simulink model "uniciclo_FL2"  (R2020a)
settings: Solver=VariableStepAuto  StartTime=0.0  StopTime=Inf  MaxStep=0.01  RelTol=1e-3
InitFcn:
  | init_biciclo
StopFcn:
  | stop_uniciclo
values from neighbouring files (symbols this model uses):
  L = 1    [init_biciclo.m]
  phi_iniziale = 0    [init_biciclo.m]
  theta_P_iniziale = pi/3    (= 1.0471975512)    [init_biciclo.m]
  v_P_dot_iniziale = 0    [init_biciclo.m]
  v_P_iniziale = 1    [init_biciclo.m]
  x_M_iniziale = 10    [init_biciclo.m]
  y_M_iniziale = -20    [init_biciclo.m]
undefined symbols (not defined in the file or in its folder): a, indexclot, Lsofar, Lsofarclot, n_p, s_f, t_f, theta_rette, v, v_raggiunta, xp, yp
libraries: simulink x1
settings Model: Creator=Andrea_Ferroni  LastModifiedBy=Andrea_Ferroni

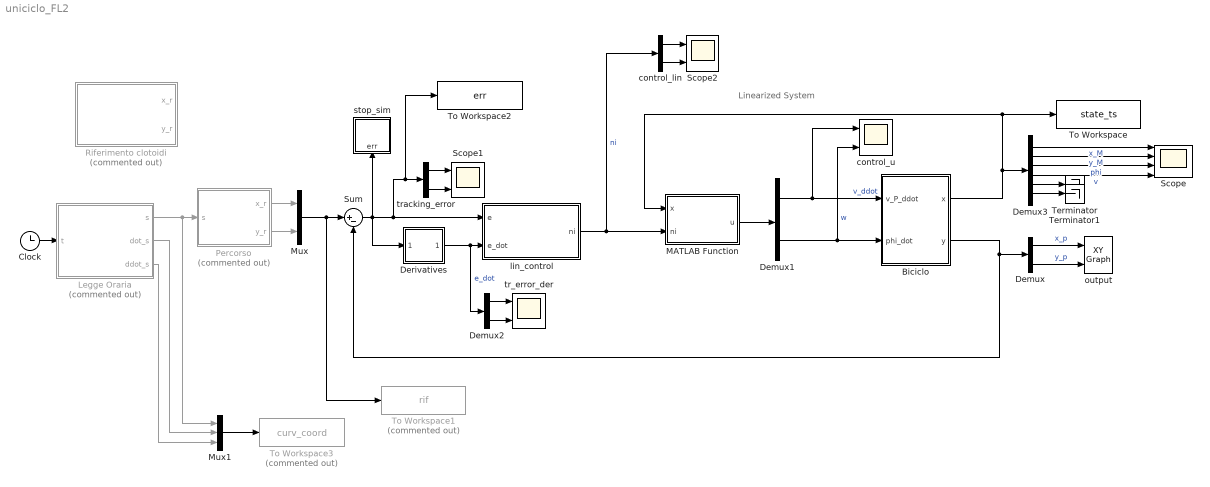
== system uniciclo_FL2 ==
  note: Linearized System
  Biciclo : Subsystem
  Clock : Clock
  Demux : Demux  Outputs=2
  Demux1 : Demux  Outputs=2
  Demux2 : Demux  Outputs=2
  Demux3 : Demux  Outputs=6
  Derivatives : Subsystem
  Legge Oraria : MATLAB Function  Commented=on  TreatAsAtomicUnit=on
  MATLAB Function : MATLAB Function  TreatAsAtomicUnit=on
  Mux : Mux  Inputs=2
  Mux1 : Mux  Inputs=3
  Percorso : MATLAB Function  Commented=on  TreatAsAtomicUnit=on
  Riferimento clotoidi : Subsystem  Commented=on
  Scope : Scope  NumInputPorts=4
  Scope1 : Scope  NumInputPorts=2
  Scope2 : Scope  NumInputPorts=2
  Sum : Sum  Inputs=|+-
  Terminator : Terminator
  Terminator1 : Terminator
  To Workspace : ToWorkspace  VariableName=state_ts  SaveFormat=Timeseries  SampleTime=-1
  To Workspace1 : ToWorkspace  Commented=on  VariableName=rif  SaveFormat=Timeseries  SampleTime=-1
  To Workspace2 : ToWorkspace  VariableName=err  SaveFormat=Timeseries  SampleTime=-1
  To Workspace3 : ToWorkspace  Commented=on  VariableName=curv_coord  SaveFormat=Timeseries  SampleTime=-1
  control_lin : Demux  Outputs=2
  control_u : Scope  NumInputPorts=2
  lin_control : MATLAB Function  TreatAsAtomicUnit=on
  output : simulink/Sinks/XY Graph  xmin=-50  xmax=50  ymin=-50  ymax=50  st=-1
  stop_sim : Subsystem
  tr_error_der : Scope  NumInputPorts=2
  tracking_error : Demux  Outputs=2
  wires:
  Biciclo/1(x) -> To Workspace/1, MATLAB Function/1(x), Demux3/1
  Mux/1 -> Sum/1, To Workspace1/1
  Biciclo/2(y) -> Demux/1, Sum/2
  lin_control/1(ni) -> control_lin/1, MATLAB Function/2(ni)  "ni"
  Sum/1 -> Derivatives/1(In1), lin_control/1(e), To Workspace2/1, tracking_error/1, stop_sim/1(err)
  Derivatives/1(Out1) -> Demux2/1, lin_control/2(e_dot)  "e_dot"
  Demux/1 -> output/1  "x_p"
  Demux/2 -> output/2  "y_p"
  Demux2/1 -> tr_error_der/1
  Demux2/2 -> tr_error_der/2
  tracking_error/1 -> Scope1/1
  tracking_error/2 -> Scope1/2
  MATLAB Function/1(u) -> Demux1/1
  Demux1/1 -> control_u/1, Biciclo/1(v_P_ddot)  "v_ddot"
  Demux1/2 -> control_u/2, Biciclo/2(phi_dot)  "w"
  control_lin/2 -> Scope2/2
  control_lin/1 -> Scope2/1
  Demux3/1 -> Scope/1  "x_M"
  Demux3/2 -> Scope/2  "y_M"
  Demux3/3 -> Scope/3  "phi"
  Demux3/4 -> Scope/4  "v"
  Clock/1 -> Legge Oraria/1(t)
  Legge Oraria/1(s) -> Mux1/1, Percorso/1(s)
  Percorso/1(x_r) -> Mux/1
  Percorso/2(y_r) -> Mux/2
  Mux1/1 -> To Workspace3/1
  Legge Oraria/3(ddot_s) -> Mux1/3
  Legge Oraria/2(dot_s) -> Mux1/2
  Demux3/6 -> Terminator1/1
  Demux3/5 -> Terminator/1

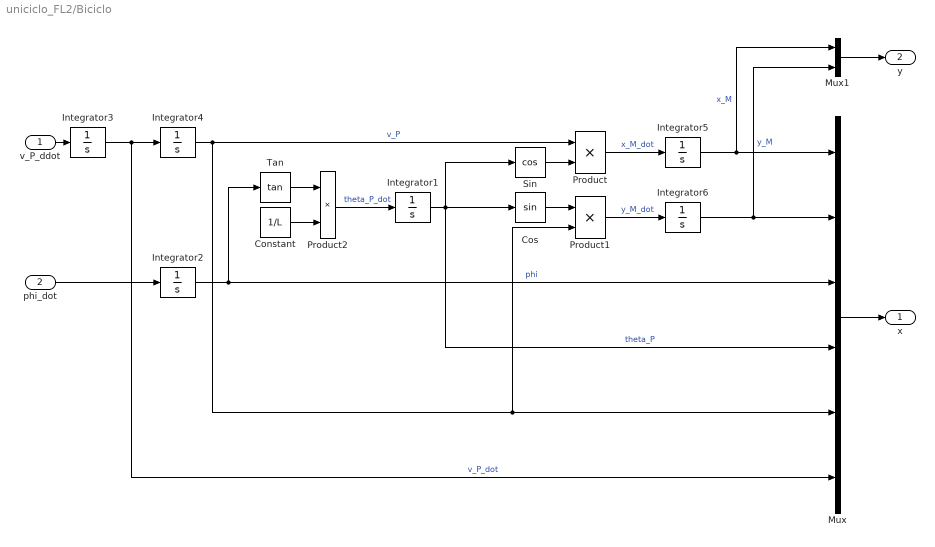
== system uniciclo_FL2/Biciclo ==
  v_P_ddot : Inport
  phi_dot : Inport  Port=2
  Constant : Constant  Value=1/L
  Cos : Trigonometry
  Integrator1 : Integrator  InitialCondition=theta_P_iniziale
  Integrator2 : Integrator  InitialCondition=phi_iniziale
  Integrator3 : Integrator  InitialCondition=v_P_dot_iniziale
  Integrator4 : Integrator  InitialCondition=v_P_iniziale
  Integrator5 : Integrator  InitialCondition=x_M_iniziale
  Integrator6 : Integrator  InitialCondition=y_M_iniziale
  Mux : Mux  Inputs=6
  Mux1 : Mux  Inputs=2
  Product : Product
  Product1 : Product
  Product2 : Product
  Sin : Trigonometry  Operator=cos
  Tan : Trigonometry  Operator=tan
  x : Outport
  y : Outport  Port=2
  wires:
  v_P_ddot/1 -> Integrator3/1
  phi_dot/1 -> Integrator2/1
  Mux/1 -> x/1
  Integrator3/1 -> Integrator4/1, Mux/6  "v_P_dot"
  Integrator1/1 -> Sin/1, Mux/4, Cos/1  "theta_P"
  Integrator4/1 -> Product1/2, Mux/5, Product/1  "v_P"
  Integrator2/1 -> Tan/1, Mux/3  "phi"
  Sin/1 -> Product/2
  Cos/1 -> Product1/1
  Product/1 -> Integrator5/1  "x_M_dot"
  Product1/1 -> Integrator6/1  "y_M_dot"
  Tan/1 -> Product2/1
  Constant/1 -> Product2/2
  Product2/1 -> Integrator1/1  "theta_P_dot"
  Mux1/1 -> y/1
  Integrator5/1 -> Mux1/1, Mux/1  "x_M"
  Integrator6/1 -> Mux1/2, Mux/2  "y_M"

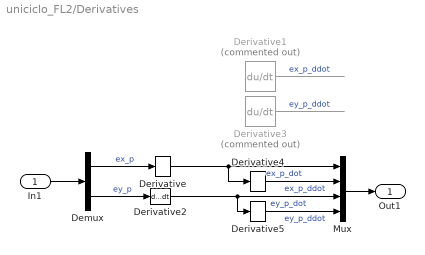
== system uniciclo_FL2/Derivatives ==
  In1 : Inport
  Demux : Demux  Outputs=2
  Derivative{,2,4..5} (4 alike) : Derivative  CoefficientInTFapproximation=1e10
  Derivative1 : Derivative  Commented=on  CoefficientInTFapproximation=1e10
  Derivative3 : Derivative  Commented=on  CoefficientInTFapproximation=1e10
  Mux : Mux
  Out1 : Outport
  wires:
  In1/1 -> Demux/1
  Demux/1 -> Derivative/1  "ex_p"
  Derivative/1 -> Derivative4/1, Mux/1  "ex_p_dot"
  Demux/2 -> Derivative2/1  "ey_p"
  Derivative1/1 -> ?  "ex_p_ddot"
  Derivative3/1 -> ?  "ey_p_ddot"
  Mux/1 -> Out1/1
  Derivative4/1 -> Mux/2  "ex_p_ddot"
  Derivative2/1 -> Derivative5/1, Mux/3  "ey_p_dot"
  Derivative5/1 -> Mux/4  "ey_p_ddot"

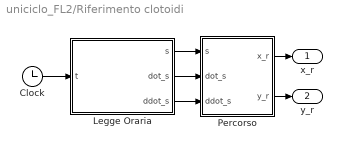
== system uniciclo_FL2/Riferimento clotoidi ==
  Clock : Clock
  Legge Oraria : MATLAB Function  TreatAsAtomicUnit=on
  Percorso : MATLAB Function  TreatAsAtomicUnit=on
  x_r : Outport
  y_r : Outport  Port=2
  wires:
  Clock/1 -> Legge Oraria/1(t)
  Legge Oraria/2(dot_s) -> Percorso/2(dot_s)
  Legge Oraria/1(s) -> Percorso/1(s)
  Legge Oraria/3(ddot_s) -> Percorso/3(ddot_s)
  Percorso/1(x_r) -> x_r/1
  Percorso/2(y_r) -> y_r/1

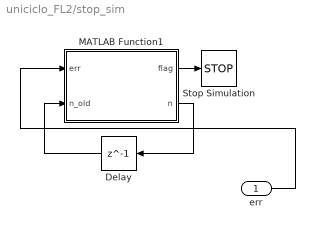
== system uniciclo_FL2/stop_sim ==
  err : Inport
  Delay : Delay  DelayLength=1
  MATLAB Function1 : MATLAB Function  TreatAsAtomicUnit=on
  Stop Simulation : Stop
  wires:
  MATLAB Function1/2(n) -> Delay/1
  MATLAB Function1/1(flag) -> Stop Simulation/1
  err/1 -> MATLAB Function1/1(err)
  Delay/1 -> MATLAB Function1/2(n_old)

== matlab function uniciclo_FL2/lin_control ==
  data: e input; ni output; e_dot input
function ni = lin_control(e, e_dot)%, K1, K2

% ni = K1.*e + K2.*e_dot;

ni = [0;0];
end

== matlab function uniciclo_FL2/MATLAB Function ==
  data: x input; ni input; u output; L parameter
function u = Linearized(x,ni,L)
E_inv = inv_E(x,L);
G = Gamma(x,L);
u =  -E_inv*G + E_inv*ni;
end

% gamma
function Gm = Gamma(x,L)
phi = x(3);
theta_P = x(4);
v_P = x(5);
v_dot = x(6);
Gm = [- (v_P*tan(phi)*((cos(theta_P)*tan(phi)*v_P^2)/L + v_dot*sin(theta_P)))/L - (2*v_P*v_dot*tan(phi)*sin(theta_P))/L;...
		(v_P*tan(phi)*(v_dot*cos(theta_P) - (v_P^2*tan(phi)*sin(theta_P))/L))/L + (2*v_P*v_dot*cos(theta_P)*tan(phi))/L];
end
% 
function E_in = inv_E(x,L)
phi = x(3);
theta_P = x(4);
v_P = x(5);
E =[ cos(theta_P), -(v_P^2*sin(theta_P)*(tan(phi)^2 + 1))/L;...
    sin(theta_P),  (v_P^2*cos(theta_P)*(tan(phi)^2 + 1))/L];
E_in = inv(E);
end

== matlab function uniciclo_FL2/Riferimento clotoidi/Legge Oraria ==
  data: t input; s output; dot_s output; ddot_s output; v_iniziale parameter
function [s, dot_s, ddot_s] = legge_oraria(t,v_iniziale)
%#codegen PEPO

s = v_iniziale*t;
dot_s = v_iniziale;
ddot_s = 0.0;

%     if v_raggiunta==0
%         
%         if t<=(s_f/a)^0.5               %acce
%             s= 0.5*a*t^2;
%             dot_s=a*t;
%             ddot_s=a;
%             
%         elseif t>(s_f/a)^0.5 & t<=t_f   %decel
%             s=s_f-0.5*a*(t_f-t)^2;
%             dot_s=-a*t;
%             ddot_s=-a;
%             
%         end
%     
%     else    
%         
%         if t<=v/a                       %acc
%             s=0.5*a*t^2;
%             dot_s=a*t;
%             ddot_s=a;
%             
%         elseif t>v/a & t<=t_f-v/a       %v=cost
%             s=0.5*a*(v/a)^2 + v *(t-v/a);
%             dot_s=v;
%             ddot_s=0;
%             
%         elseif t>t_f-v/a & t<=t_f       %decel
%             s=s_f-0.5*a*(t_f-t)^2;
%             dot_s=v-a*(t - (t_f-v/a));
%             ddot_s=-a;
%             
%             
%         end
%             
%     end

end

== matlab function uniciclo_FL2/stop_sim/MATLAB Function1 ==
  data: flag output; err input; n output; n_old input; threshold parameter
function [flag, n] = stop_function(err, n_old, threshold)
	flag = 0;
	n = n_old;
	if norm(err, 2) < threshold
		n=n+1;
	else
		n=0;
	end
	
	if n > 10
		flag = 1;
		n = 0;
	end
end

== matlab function uniciclo_FL2/Riferimento clotoidi/Percorso ==
  data: s input; x_r output; dot_s input; ddot_s input; y_r output; a parameter; indexclot parameter; Lsofar parameter; Lsofarclot parameter; n_p parameter; s_f parameter; t_f parameter; theta_rette parameter; v parameter; v_raggiunta parameter; xp parameter; yp parameter
function [x_r,y_r ] = percorso(s, dot_s,ddot_s, a, indexclot, Lsofar, Lsofarclot, n_p, s_f, t_f, theta_rette, v, v_raggiunta, xp, yp)
%#codegen      PEPO


coder.extrinsic('pointsOnClothoid')

% v_r = dot_s ;
ntratto=0;
XYS=[0 0]'; %definito prima
%clot=struct('x0', 0, 'y0', 0, 'theta0', 0 , 'k0', 0, 'dk', 0, 'L', 0 );

%Parte per capire in che tratto sono
    if s<Lsofar(1)
        ntratto=1;
    else
    	for ii=2:(n_p-1)
        	if s>=Lsofar(ii-1) && s<=Lsofar(ii)
                ntratto=ii;
            end
    	end
    end

    
    
%calcolo delle coordinate x e y riferite a s e a ntratto
    if mod(ntratto,2)==1            %tratti dispari
        if ntratto==1
            XYS=[xp(ntratto)+cos(theta_rette(ntratto))*(s), yp(ntratto)+sin(theta_rette(ntratto))*(s)]';
        else
            XYS=[xp(ntratto)+cos(theta_rette(ntratto))*(s-Lsofar(ntratto-1)), yp(ntratto)+sin(theta_rette(ntratto))*(s-Lsofar(ntratto-1))]';
        end 

    elseif mod(ntratto,2)==0
        srel=s-Lsofar(ntratto-1);
        
        
        if srel<=Lsofarclot(ntratto/2).Lclot(1)
            XYS = double(pointsOnClothoid( indexclot(ntratto/2).clot.S0, srel ));
            
        elseif srel>Lsofarclot(ntratto/2).Lclot(1) & srel<=Lsofarclot(ntratto/2).Lclot(2)
            XYS = double(pointsOnClothoid( indexclot(ntratto/2).clot.SM, srel- indexclot(ntratto/2).clot.S0.L ));
            
        elseif srel>Lsofarclot(ntratto/2).Lclot(2)
            XYS = double(pointsOnClothoid( indexclot(ntratto/2).clot.S1, srel- indexclot(ntratto/2).clot.S0.L - indexclot(ntratto/2).clot.SM.L ));
        end
        
        
        
        %XYS = double(pointsOnClothoid( indexclot(ntratto/2).clot, s-Lsofar(ntratto-1) ));
        
    end

    x_r=XYS(1);
    y_r=XYS(2);

end

== matlab function uniciclo_FL2/Legge Oraria ==
  data: t input; s output; v_rif parameter; dot_s output; ddot_s output
function [s, dot_s, ddot_s]  = legge_oraria(t, v_rif)
%#codegen PEPO

s = v_rif*t;
dot_s = v_rif;
ddot_s = 0.0;

%     if v_raggiunta==0
%         
%         if t<=(s_f/a)^0.5               %acce
%             s= 0.5*a*t^2;
%             dot_s=a*t;
%             ddot_s=a;
%             
%         elseif t>(s_f/a)^0.5 & t<=t_f   %decel
%             s=s_f-0.5*a*(t_f-t)^2;
%             dot_s=-a*t;
%             ddot_s=-a;
%             
%         end
%     
%     else    
%         
%         if t<=v/a                       %acc
%             s=0.5*a*t^2;
%             dot_s=a*t;
%             ddot_s=a;
%             
%         elseif t>v/a & t<=t_f-v/a       %v=cost
%             s=0.5*a*(v/a)^2 + v *(t-v/a);
%             dot_s=v;
%             ddot_s=0;
%             
%         elseif t>t_f-v/a & t<=t_f       %decel
%             s=s_f-0.5*a*(t_f-t)^2;
%             dot_s=v-a*(t - (t_f-v/a));
%             ddot_s=-a;
%             
%             
%         end
%             
%     end

end

== matlab function uniciclo_FL2/Percorso ==
  data: s input; x_r output; y_r output
function [x_r, y_r] = percorso(s)



% pos = s * [0; 1] + [1; 0]*cos(s);				% sinusoide

r = 10;
theta_circ = s/r;

pos = r*[cos(theta_circ);sin(theta_circ)];		% circonferenza
%p = [cos(s/2);sin(s/2)];
%pos = min(1/(s/100+0.01),r) * p;					% spirale
%pos = 1/(s/100+0.01) * p;

x_r = pos(1);
y_r = pos(2);

end
